simulink model "TVsimModelnoCA"  (R2023a)
settings: Solver=ode4  StartTime=0.0  StopTime=10.0  FixedStep=0.001  RelTol=1e-3
values from neighbouring files (symbols this model uses):
  K_att1 = lqr(AA,BA,QA,RA)    [controllerParams.m]
  K_att2 = inv(BA'*BA)*BA'*AA    [controllerParams.m]
  K_pos1 = lqr(AP,BP,QP,RP)    [controllerParams.m]
  K_pos2 = inv(BP'*BP)*BP'*AP    [controllerParams.m]
  x0 = [0,0,0,0,0,0,0,0,0,0,0,0]'    [TVquadTrackingProblem.m]    (also in runTVTrackingProblemCA.m; thrustVectoringQuadTrackingProblem.m = [0,0,0,0,0,0,0,0,0.2,0,0,0]')
undefined symbols (not defined in the file or in its folder): TVequationsOfMotion
settings Model: Creator=Jann-AIMLAB  LastModifiedBy=Jann-AIMLAB

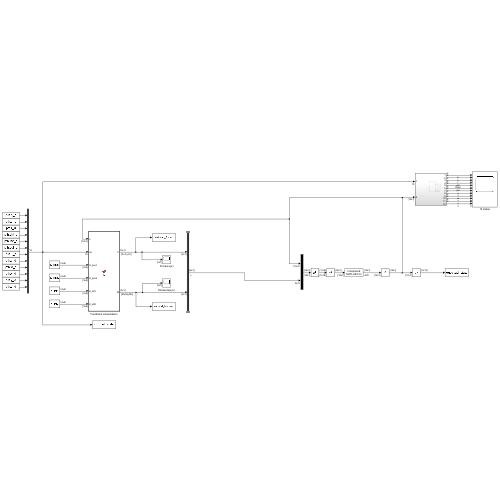
[thumbnail: Simulink's stored preview of the top-level diagram]
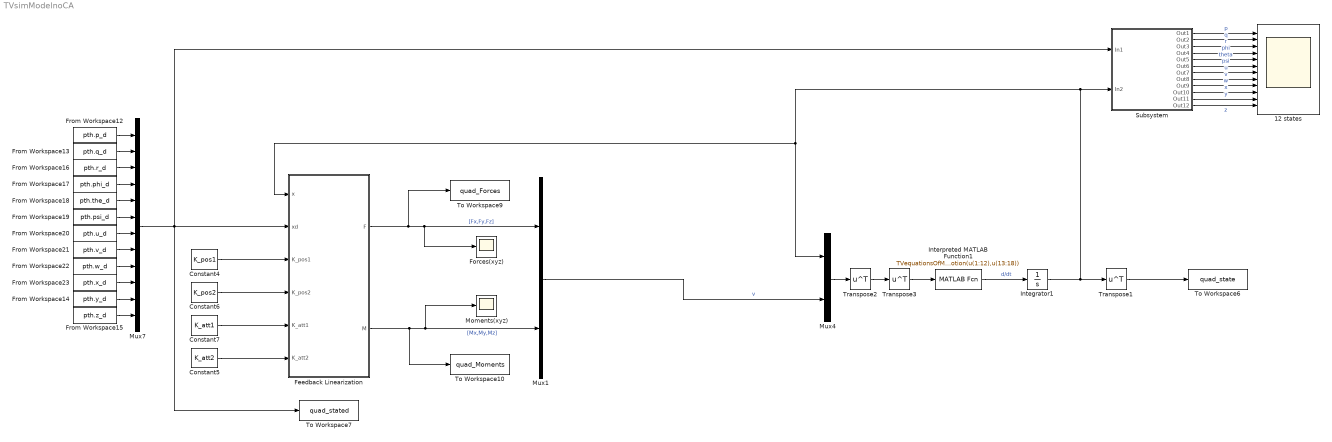
== system TVsimModelnoCA ==
  12 states : Scope  NumInputPorts=12
  Constant4 : Constant  Value=K_pos1  VectorParams1D=off
  Constant5 : Constant  Value=K_att2  VectorParams1D=off
  Constant6 : Constant  Value=K_pos2  VectorParams1D=off
  Constant7 : Constant  Value=K_att1  VectorParams1D=off
  Feedback Linearization : MATLAB Function  TreatAsAtomicUnit=on
  Forces(xyz) : Scope
  From Workspace12 : FromWorkspace  VariableName=pth.p_d
  From Workspace13 : FromWorkspace  VariableName=pth.q_d
  From Workspace14 : FromWorkspace  VariableName=pth.y_d
  From Workspace15 : FromWorkspace  VariableName=pth.z_d
  From Workspace16 : FromWorkspace  VariableName=pth.r_d
  From Workspace17 : FromWorkspace  VariableName=pth.phi_d
  From Workspace18 : FromWorkspace  VariableName=pth.the_d
  From Workspace19 : FromWorkspace  VariableName=pth.psi_d
  From Workspace20 : FromWorkspace  VariableName=pth.u_d
  From Workspace21 : FromWorkspace  VariableName=pth.v_d
  From Workspace22 : FromWorkspace  VariableName=pth.w_d
  From Workspace23 : FromWorkspace  VariableName=pth.x_d
  Integrator1 : Integrator  InitialCondition=x0
  Interpreted MATLAB Function1 : MATLABFcn  MATLABFcn=TVequationsOfMotion(u(1:12),u(13:18))  Output1D=off
  Moments(xyz) : Scope
  Mux1 : Mux  Inputs=2
  Mux4 : Mux  Inputs=2
  Mux7 : Mux  Inputs=12
  Subsystem : Subsystem
  To Workspace10 : ToWorkspace  VariableName=quad_Moments  SaveFormat=Timeseries  SampleTime=-1
  To Workspace6 : ToWorkspace  VariableName=quad_state  SampleTime=-1
      settings: Save2DSignal=2-D array (concatenate along first dimension)
  To Workspace7 : ToWorkspace  VariableName=quad_stated  SaveFormat=Timeseries  SampleTime=-1
  To Workspace9 : ToWorkspace  VariableName=quad_Forces  SaveFormat=Timeseries  SampleTime=-1
  Transpose1 : Math  Operator=transpose
  Transpose2 : Math  Operator=transpose
  Transpose3 : Math  Operator=transpose
  wires:
  Mux4/1 -> Transpose2/1
  From Workspace17/1 -> Mux7/4
  Subsystem/2(Out2) -> 12 states/2  "q"
  Subsystem/12(Out12) -> 12 states/12  "z"
  Subsystem/4(Out4) -> 12 states/4  "phi"
  From Workspace21/1 -> Mux7/8
  From Workspace16/1 -> Mux7/3
  Integrator1/1 -> Subsystem/2(In2), Feedback Linearization/1(x), Mux4/1, Transpose1/1
  From Workspace12/1 -> Mux7/1
  From Workspace22/1 -> Mux7/9
  From Workspace18/1 -> Mux7/5
  From Workspace13/1 -> Mux7/2
  Constant5/1 -> Feedback Linearization/6(K_att2)
  Subsystem/1(Out1) -> 12 states/1  "p"
  Constant4/1 -> Feedback Linearization/3(K_pos1)
  Feedback Linearization/2(M) -> To Workspace10/1, Mux1/2, Moments(xyz)/1  "[Mx,My,Mz]"
  Subsystem/5(Out5) -> 12 states/5  "theta"
  From Workspace23/1 -> Mux7/10
  From Workspace15/1 -> Mux7/12
  From Workspace19/1 -> Mux7/6
  Interpreted MATLAB Function1/1 -> Integrator1/1  "d/dt"
  From Workspace14/1 -> Mux7/11
  Mux7/1 -> Subsystem/1(In1), Feedback Linearization/2(xd), To Workspace7/1
  Constant6/1 -> Feedback Linearization/4(K_pos2)
  Subsystem/8(Out8) -> 12 states/8  "v"
  Constant7/1 -> Feedback Linearization/5(K_att1)
  Subsystem/3(Out3) -> 12 states/3  "r"
  Transpose3/1 -> Interpreted MATLAB Function1/1
  Feedback Linearization/1(F) -> To Workspace9/1, Mux1/1, Forces(xyz)/1  "[Fx,Fy,Fz]"
  Transpose2/1 -> Transpose3/1
  Subsystem/10(Out10) -> 12 states/10  "x"
  Subsystem/9(Out9) -> 12 states/9  "w"
  Subsystem/6(Out6) -> 12 states/6  "psi"
  Subsystem/11(Out11) -> 12 states/11  "y"
  Subsystem/7(Out7) -> 12 states/7  "u"
  Transpose1/1 -> To Workspace6/1
  From Workspace20/1 -> Mux7/7
  Mux1/1 -> Mux4/2  "v"

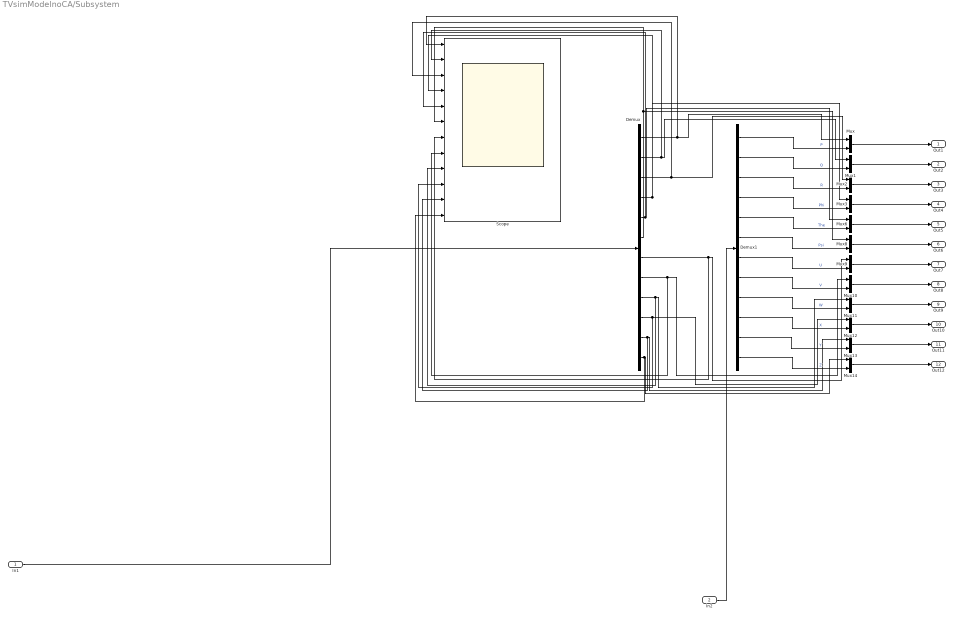
== system TVsimModelnoCA/Subsystem ==
  In1 : Inport
  In2 : Inport  Port=2
  Demux : Demux  Outputs=12
  Demux1 : Demux  Outputs=12
  Mux{,1..3,6,8..14} (12 alike) : Mux  Inputs=2
  Scope : Scope  NumInputPorts=12
  Out1 : Outport
  Out2 : Outport  Port=2
  Out3 : Outport  Port=3
  Out4 : Outport  Port=4
  Out5 : Outport  Port=5
  Out6 : Outport  Port=6
  Out7 : Outport  Port=7
  Out8 : Outport  Port=8
  Out9 : Outport  Port=9
  Out10 : Outport  Port=10
  Out11 : Outport  Port=11
  Out12 : Outport  Port=12
  wires:
  Demux/9 -> Scope/9, Mux11/1
  Demux1/9 -> Mux11/2  "W"
  Demux/7 -> Scope/7, Mux9/1
  In2/1 -> Demux1/1
  Demux1/5 -> Mux6/2  "The"
  Demux1/10 -> Mux12/2  "X"
  Demux1/2 -> Mux1/2  "Q"
  Demux1/7 -> Mux9/2  "U"
  Mux10/1 -> Out8/1
  Demux1/11 -> Mux13/2  "Y"
  Demux/3 -> Scope/3, Mux2/1
  Demux/11 -> Scope/11, Mux13/1
  Demux1/8 -> Mux10/2  "V"
  Mux2/1 -> Out3/1
  Demux/6 -> Scope/6, Mux8/1
  Demux1/4 -> Mux3/2  "Phi"
  Demux/5 -> Scope/5, Mux6/1
  Demux/8 -> Scope/8, Mux10/1
  Demux1/1 -> Mux/2  "P"
  Demux/10 -> Scope/10, Mux12/1
  Mux8/1 -> Out6/1
  Demux1/3 -> Mux2/2  "R"
  Demux/1 -> Scope/1, Mux/1
  Demux1/6 -> Mux8/2  "Psi"
  Mux11/1 -> Out9/1
  Demux1/12 -> Mux14/2  "Z"
  Mux6/1 -> Out5/1
  Mux/1 -> Out1/1
  Demux/12 -> Scope/12, Mux14/1
  Demux/2 -> Scope/2, Mux1/1
  Mux12/1 -> Out10/1
  Demux/4 -> Scope/4, Mux3/1
  Mux13/1 -> Out11/1
  Mux3/1 -> Out4/1
  In1/1 -> Demux/1
  Mux14/1 -> Out12/1
  Mux9/1 -> Out7/1
  Mux1/1 -> Out2/1

== matlab function TVsimModelnoCA/Feedback Linearization ==
  data: x input; F output; xd input; K_pos1 input; M output; K_pos2 input; K_att1 input; K_att2 input
function [F,M] = fbl(x,xd,K_pos1,K_pos2,K_att1,K_att2)
% CALCULATE MOMENT AND THRUST FORCES
%find k,d,l
k=2.98e-06; kQ = 1.14e-7;%kQ=.0382; 
%find m,Ixx,Iyy,Izz,Ir
m=0.468; 
%m = 0.68;
g = 9.81;
Ixx=4.856e-03;Iyy=4.856e-03;Izz=8.801e-03;

Ir=3.357e-05;
Ax=.3; Ay=0.3; Az=0.25; Ar=0.2;

Omega =0;

%Omega = w(1)-w(2)+w(3)-w(4);   
% if size(w) == [1,1]
% Omega = 0;
% else
% Omega = w(1)-w(2)+w(3)-w(4);
% end


% states: x = [p,q,r,phi,the,psi,u,v,w,x,y,z];

% position control
% state error 
e_p = x(7:12) - xd(7:12);
% f_p = -(1/m)*[Ax,0,0,0,0,0;
%                0,Ay,0,0,0,0;
%                0,0,Az + g,0,0,0;
%                1,0,0,0,0,0;
%                0,1,0,0,0,0;
%                0,0,1,0,0,0];
f_p = [-(1/m)*(Ax*x(7));
    -(1/m)*(Ay*x(8));
    -(1/m)*(Az*x(9));
    x(7);
    x(8);
    x(9)];
g_p = (1/m)*[cos(x(6))*cos(x(5)), cos(x(4))*sin(x(6)) + cos(x(6))*sin(x(4))*sin(x(5)), sin(x(4))*sin(x(6)) - cos(x(4))*cos(x(6))*sin(x(5)), 0, 0, 0;
					-cos(x(5))*sin(x(6)), cos(x(4))*cos(x(6)) - sin(x(4))*sin(x(6))*sin(x(5)), cos(x(6))*sin(x(4)) + cos(x(4))*sin(x(6))*sin(x(5)), 0, 0, 0;
					sin(x(5)), -cos(x(5))*sin(x(4)), cos(x(4))*cos(x(5)), 0, 0, 0;
					0,0,0,0,0,0;
					0,0,0,0,0,0;
					0,0,0,0,0,0];

% F = g_p(1:3,1:3)\(-(f_p(4:6).'*f_p(1:3))-10.*K_pos1*e_p-0.*K_pos2*xd(7:12));
%F = m.*(-(f_p(4:6).'*f_p(1:3))-K_pos1*e_p-K_pos2*xd(7:12));
F = g_p(1:3,1:3)\(-(f_p(4:6).'*f_p(1:3))-K_pos1*e_p);

% attitude control 
e_a = x(1:6) - xd(1:6);
f_a = [(1/Ixx)*((Iyy-Izz)*x(2)*x(3)-Ir*x(2)*Omega-Ar*x(1));
    (1/Iyy)*((Ixx-Izz)*x(1)*x(3)-Ir*x(1)*Omega-Ar*x(2));
    (1/Izz)*((Iyy-Ixx)*x(2)*x(1)-Ar*x(3));
    x(1) + sin(x(4))*tan(x(5))*x(2) + cos(x(4))*tan(x(5))*x(3);
    cos(x(4))*x(2) - sin(x(4))*x(3);
    sin(x(4))/cos(x(5))*x(2) + cos(x(4))/cos(x(5))*x(3)];
g_a = [(1/Ixx),0,0,0,0,0;
    0,(1/Iyy),0,0,0,0;
    0,0,(1/Izz),0,0,0;
    0,0,0,0,0,0;
    0,0,0,0,0,0;
    0,0,0,0,0,0];

%M = g_a(1:3,1:3)\(-(f_a(4:6).'*f_a(1:3))-10.*K_att1*e_a-0.*K_att2*xd(1:6));
M = g_a(1:3,1:3)\(-(f_a(4:6).'*f_a(1:3))-K_att1*e_a);
